simulink model "SSN2"  (Simulink 7.6)
settings: Solver=FixedStepDiscrete  StartTime=0.0  StopTime=10.0  FixedStep=0.5  RelTol=1e-3
libraries: xpclib x1
(part 1 of 3)
settings Model: Creator=jdethier  LastModifiedBy=jdethier  SimulationMode=external  BufferReuse=off
settings OptimizationCC: BlockReduction=off  OptimizeBlockIOStorage=off  BufferReuse=off  ExpressionFolding=off  LocalBlockOutputs=off
settings HardwareCC: ProdIntDivRoundTo=Zero  ProdEndianess=LittleEndian  ProdHWDeviceType=Generic->32-bit x86 compatible
settings RTWCC: SystemTargetFile=xpctarget.tlc  TemplateMakefile=xpc_default_tmf  Description=xPC Target  ProcessScript=xpctarget_make_rtw_hook  RTWCompilerOptimization=On
settings xpcTargetCC: TargetFcnLib=ansi_tfl_table_tmw.mat  TargetFunctionLibrary=XPC_BLAS  ERTCodeCoverageTool=None  ParMdlRefBuildCompliant=on  CombineSignalStateStructs=off  PortableWordSizes=off  xPCLoadParamSetFile=off  xPCConcurrentTasks=off  xPCEnableSFAnimation=off

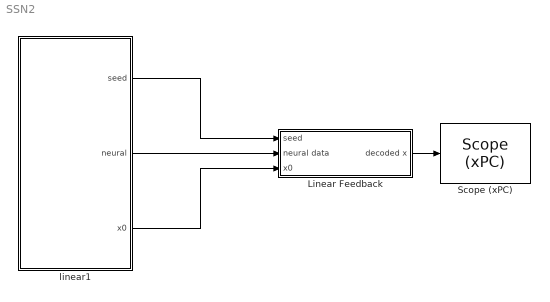
== system SSN2 ==
  Linear Feedback : Subsystem
  "Scope (xPC) " : xpclib/Misc./Scope (xPC)   SystemSampleTime=-1  scopeno=1  scopetype=Target  autostart=on  viewmode=Numerical  formatstr='%15.6f'  grid=on  ylimits=[0,0]  nosamples=3  noprepostsamples=0  interleave=1  triggermode=FreeRun  triggersignal=1  triggerlevel=0.0  triggerslope=Either  triggerscope=1  triggersample=0  filename=data.dat  mode=Lazy  writesize=512  autorestart=off  dynamicfilemode=off  maxwritefilesize=512*1024^2
  linear1 : Stateflow chart  TreatAsAtomicUnit=on
  wires:
  linear1/1(seed) -> Linear Feedback/1(seed)
  linear1/2(neural) -> Linear Feedback/2(neural data)
  linear1/3(x0) -> Linear Feedback/3(x0)
  Linear Feedback/1(decoded x) -> "Scope (xPC) "/1

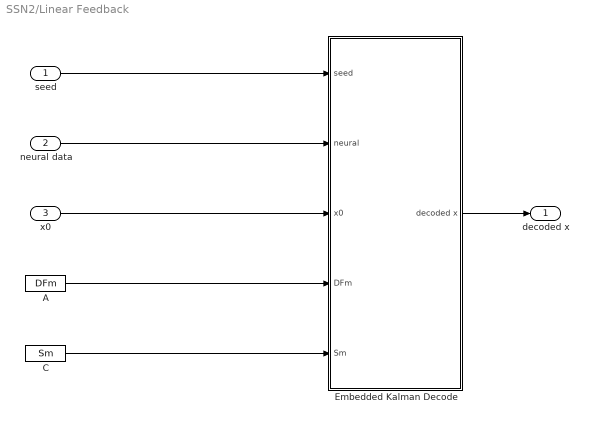
== system SSN2/Linear Feedback ==
  seed : Inport
  neural data : Inport  Port=2
  x0 : Inport  Port=3
  A : FromWorkspace  VariableName=DFm  Interpolate=off  OutputAfterFinalValue=Holding final value
  C : FromWorkspace  VariableName=Sm  Interpolate=off  OutputAfterFinalValue=Holding final value
  Embedded Kalman Decode : Subsystem
  decoded x : Outport
  wires:
  A/1 -> Embedded Kalman Decode/4(DFm)
  C/1 -> Embedded Kalman Decode/5(Sm)
  neural data/1 -> Embedded Kalman Decode/2(neural)
  x0/1 -> Embedded Kalman Decode/3(x0)
  seed/1 -> Embedded Kalman Decode/1(seed)
  Embedded Kalman Decode/1(decoded x) -> decoded x/1

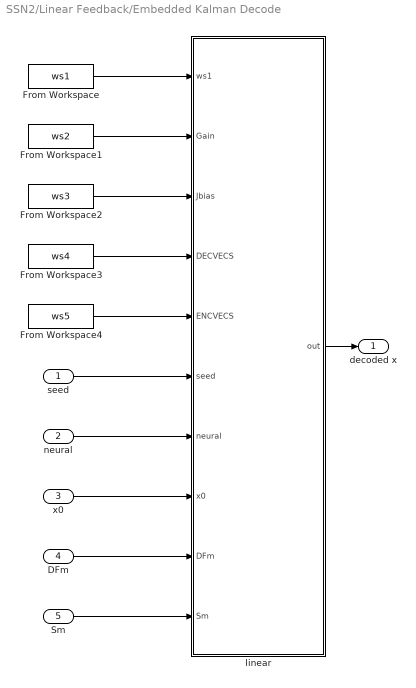
== system SSN2/Linear Feedback/Embedded Kalman Decode ==
  seed : Inport
  neural : Inport  Port=2
  x0 : Inport  Port=3
  DFm : Inport  Port=4
  Sm : Inport  Port=5
  From Workspace : FromWorkspace  VariableName=ws1  Interpolate=off  OutputAfterFinalValue=Holding final value
  From Workspace1 : FromWorkspace  VariableName=ws2  Interpolate=off  OutputAfterFinalValue=Holding final value
  From Workspace2 : FromWorkspace  VariableName=ws3  Interpolate=off  OutputAfterFinalValue=Holding final value
  From Workspace3 : FromWorkspace  VariableName=ws4  Interpolate=off  OutputAfterFinalValue=Holding final value
  From Workspace4 : FromWorkspace  VariableName=ws5  Interpolate=off  OutputAfterFinalValue=Holding final value
  linear : Stateflow chart  TreatAsAtomicUnit=on
  decoded x : Outport
  wires:
  linear/1(out) -> decoded x/1
  Sm/1 -> linear/10(Sm)
  DFm/1 -> linear/9(DFm)
  x0/1 -> linear/8(x0)
  neural/1 -> linear/7(neural)
  seed/1 -> linear/6(seed)
  From Workspace/1 -> linear/1(ws1)
  From Workspace1/1 -> linear/2(Gain)
  From Workspace2/1 -> linear/3(Jbias)
  From Workspace3/1 -> linear/4(DECVECS)
  From Workspace4/1 -> linear/5(ENCVECS)
